simulink model "PMSM"  (R2020a)
settings: Solver=ode45  StartTime=0.0  StopTime=10.0  RelTol=1e-6  AbsTol=1e-8
values from neighbouring files (symbols this model uses):
  B = 0.08    [Mainprog.m]
  Ba = alphas * Jhat - Bhat    (= 0.17)    [Mainprog.m]
  J = 0.05*0.25    (= 0.0125)    [Mainprog.m]
  kis = alphas * (Bhat + Ba)    (= 5)    [Mainprog.m]
  kps = alphas * Jhat    (= 0.25)    [Mainprog.m]
  np = 2    [Mainprog.m]
  Rs = 1.33    [Mainprog.m]
undefined symbols (not defined in the file or in its folder): Beta_initial, Beta_timeup, fluxm, fluxm_hat, i, I_rated, isd0, isq0, j, kicd, kicq, kpcd, kpcq, Lsd, Lsd_hat, Lsq, Lsq_hat, Rad, Raq, Speed_initial, Speed_timeup, Speed_valueup, T_extra_timeup, T_extra_valup, T_ref1_timeup, T_ref1_valup, T_ref2_timeup, T_ref2_valup, thetar0, usd0, usq0, VconvLim, wr0, ws
settings Model: ExtModeTrigMode=oneshot  ExtModeArmWhenConnect=off  ExtModeAutoUpdateStatusClock=off  Creator=e6zebra  LastModifiedBy=miche
settings SolverCC: AutoScaleAbsTol=off
settings DataIOCC: SaveFormat=Array  SignalLoggingSaveFormat=ModelDataLogs  ReturnWorkspaceOutputs=off
settings OptimizationCC: BlockReduction=off  BooleanDataType=off  ExpressionDepthLimit=2147483647  InitFltsAndDblsToZero=on  LifeSpan=inf
settings DebuggingCC: SaveWithParameterizedLinksMsg=none  UnderspecifiedInitializationDetection=Classic  MergeDetectMultiDrivingBlocksExec=none  SignalResolutionControl=TryResolveAllWithWarning  MultiTaskDSMMsg=warning  MultiTaskCondExecSysMsg=none  FcnCallInpInsideContextMsg=warning  StateNameClashWarn=warning  SFUnexpectedBacktrackingDiag=warning  SFNoUnconditionalDefaultTransitionDiag=warning  SFExecutionAtInitializationDiag=none  ArithmeticOperatorsInVariantConditions=warning
settings HardwareCC: ProdBitPerPointer=32  ProdBitPerSizeT=32  ProdBitPerPtrDiffT=32  ProdLargestAtomicFloat=None  ProdIntDivRoundTo=Undefined  ProdEndianess=Unspecified  ProdWordSize=32  ProdHWDeviceType=32-bit Generic  TargetUnknown=on
settings ModelReferenceCC: PropagateSignalLabelsOutOfModel=off
settings SFSimCC: SimUseLocalCustomCode=off  CustomCodeUndefinedFunction=UseInterfaceOnly
settings RTWCC: TemplateMakefile=grt.tmf  RTWUseLocalCustomCode=off
settings CodeAppCC: StateflowObjectComments=on
settings GRTTargetCC: TargetFcnLib=ansi_tfl_tmw.mat  TargetLangStandard=C89/C90 (ANSI)  CombineOutputUpdateFcns=off  GRTInterface=on
settings ConfigComp: CovMetricSettings=dw  CovHtmlReporting=on  CovSaveCumulativeToWorkspaceVar=on  CovSaveSingleToWorkspaceVar=on  CovExternalEMLEnable=off  CovSFcnEnable=off

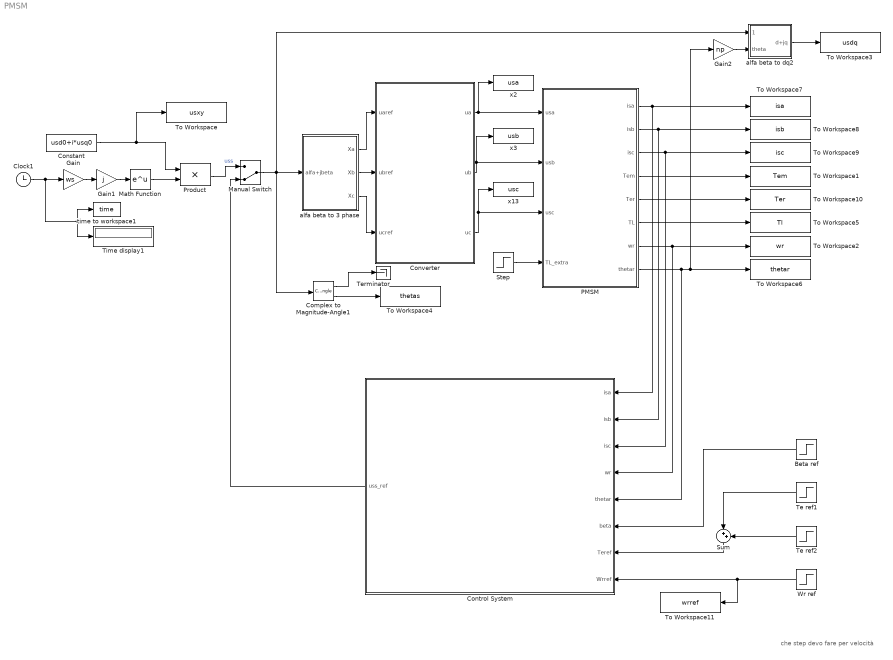
== system PMSM ==
  note: che step devo fare per velocità
  Beta ref : Step  Time=Beta_timeup  Before=Beta_initial  After=Beta_initial  SampleTime=0
  Clock1 : Clock
  Complex to Magnitude-Angle1 : ComplexToMagnitudeAngle
  Constant : Constant  Value=usd0+i*usq0
  Control System : Subsystem
  Converter : Subsystem
  Gain : Gain  Gain=ws
  Gain1 : Gain  Gain=j  SaturateOnIntegerOverflow=on  OutDataTypeStr=Inherit: Same as input  ParamDataTypeStr=Inherit: Same as input
  Gain2 : Gain  Gain=np
  Manual Switch : ManualSwitch  CurrentSetting=0
  Math Function : Math  SignedPower=on  SaturateOnIntegerOverflow=on
  PMSM : Subsystem
  Product : Product  SaturateOnIntegerOverflow=on  OutDataTypeStr=Inherit: Same as first input
  Step : Step  Time=T_extra_timeup  After=T_extra_valup  SampleTime=0
  Sum : Sum  Inputs=|++
  Te ref1 : Step  Time=T_ref1_timeup  After=T_ref1_valup  SampleTime=0
  Te ref2 : Step  Time=T_ref2_timeup  After=T_ref2_valup  SampleTime=0
  Terminator : Terminator
  Time display1 : Display
  To Workspace : ToWorkspace  VariableName=usxy  SampleTime=-1
  To Workspace1 : ToWorkspace  VariableName=Tem  SampleTime=-1
  To Workspace10 : ToWorkspace  VariableName=Ter  SampleTime=-1
  To Workspace11 : ToWorkspace  VariableName=wrref  SampleTime=-1
  To Workspace2 : ToWorkspace  VariableName=wr  SampleTime=-1
  To Workspace3 : ToWorkspace  VariableName=usdq  SampleTime=-1
  To Workspace4 : ToWorkspace  VariableName=thetas  SampleTime=-1
  To Workspace5 : ToWorkspace  VariableName=Tl  SampleTime=-1
  To Workspace6 : ToWorkspace  VariableName=thetar  SampleTime=-1
  To Workspace7 : ToWorkspace  VariableName=isa  SampleTime=-1
  To Workspace8 : ToWorkspace  VariableName=isb  SampleTime=-1
  To Workspace9 : ToWorkspace  VariableName=isc  SampleTime=-1
  Wr ref : Step  Time=Speed_timeup  Before=Speed_initial  After=Speed_valueup  SampleTime=0
  alfa beta to 3 phase : Subsystem
  alfa beta to dq2 : Subsystem
  time to workspace1 : ToWorkspace  VariableName=time  SampleTime=-1
  x13 : ToWorkspace  VariableName=usc  SampleTime=-1
  x2 : ToWorkspace  VariableName=usa  SampleTime=-1
  x3 : ToWorkspace  VariableName=usb  SampleTime=-1
  wires:
  Converter/1(ua) -> x2/1, PMSM/1(usa)
  alfa beta to 3 phase/3(Xc) -> Converter/3(ucref)
  Complex to Magnitude-Angle1/2 -> To Workspace4/1
  alfa beta to 3 phase/1(Xa) -> Converter/1(uaref)
  Gain1/1 -> Math Function/1
  Clock1/1 -> Time display1/1, time to workspace1/1, Gain/1
  alfa beta to 3 phase/2(Xb) -> Converter/2(ubref)
  Gain/1 -> Gain1/1
  Math Function/1 -> Product/2
  Complex to Magnitude-Angle1/1 -> Terminator/1
  Step/1 -> PMSM/4(TL_extra)
  Constant/1 -> To Workspace/1, Product/1
  alfa beta to dq2/1(d+jq) -> To Workspace3/1
  PMSM/8(thetar) -> Control System/5(thetar), To Workspace6/1, Gain2/1
  Gain2/1 -> alfa beta to dq2/2(theta)
  PMSM/7(wr) -> To Workspace2/1, Control System/4(wr)
  PMSM/6(TL) -> To Workspace5/1
  Converter/2(ub) -> x3/1, PMSM/2(usb)
  Converter/3(uc) -> PMSM/3(usc), x13/1
  PMSM/1(isa) -> To Workspace7/1, Control System/1(isa)
  PMSM/2(isb) -> To Workspace8/1, Control System/2(isb)
  PMSM/3(isc) -> To Workspace9/1, Control System/3(isc)
  PMSM/4(Tem) -> To Workspace1/1
  PMSM/5(Ter) -> To Workspace10/1
  Manual Switch/1 -> Complex to Magnitude-Angle1/1, alfa beta to dq2/1(alfa+jbeta), alfa beta to 3 phase/1(alfa+jbeta)
  Product/1 -> Manual Switch/1  "uss"
  Control System/1(uss_ref) -> Manual Switch/2
  Te ref1/1 -> Sum/1
  Te ref2/1 -> Sum/2
  Sum/1 -> Control System/7(Teref)
  Wr ref/1 -> To Workspace11/1, Control System/8(Wrref)
  Beta ref/1 -> Control System/6(beta)

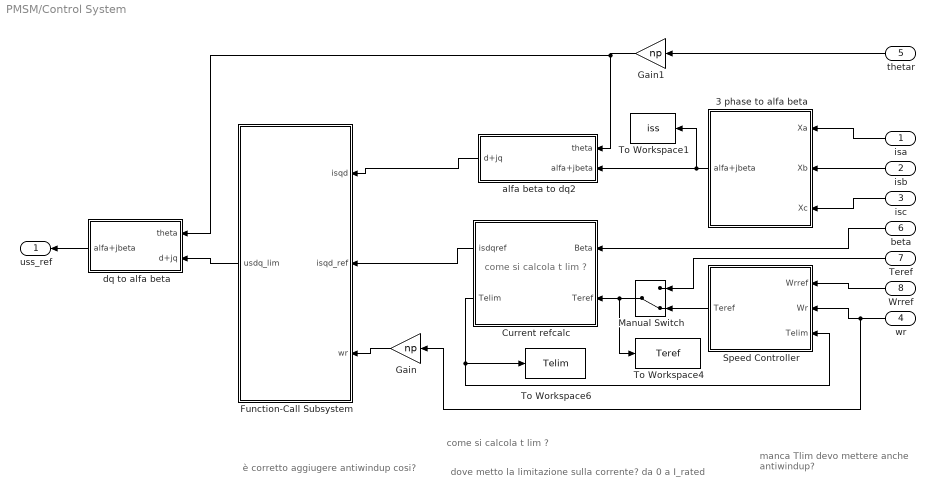
== system PMSM/Control System ==
  note: come si calcola t lim ?
  note: dove metto la limitazione sulla corrente? da 0 a I_rated
  note: è corretto aggiugere antiwindup cosi?
  note: manca Tlim
      |
      | devo mettere anche antiwindup?
  note: come si calcola t lim ?
  isa : Inport
  isb : Inport  Port=2
  isc : Inport  Port=3
  wr : Inport  Port=4
  thetar : Inport  Port=5
  beta : Inport  Port=6
  Teref : Inport  Port=7
  Wrref : Inport  Port=8
  3 phase to alfa beta : Subsystem
  Current refcalc : Subsystem
  Function-Call Subsystem : Subsystem  TreatAsAtomicUnit=on
  Gain : Gain  Gain=np
  Gain1 : Gain  Gain=np
  Manual Switch : ManualSwitch  CurrentSetting=0
  Speed Controller : Subsystem
  To Workspace1 : ToWorkspace  VariableName=iss  SampleTime=-1
  To Workspace4 : ToWorkspace  VariableName=Teref  SampleTime=-1
  To Workspace6 : ToWorkspace  VariableName=Telim  SampleTime=-1
  alfa beta to dq2 : Subsystem
  dq to alfa beta : Subsystem
  uss_ref : Outport
  wires:
  dq to alfa beta/1(alfa+jbeta) -> uss_ref/1
  alfa beta to dq2/1(d+jq) -> Function-Call Subsystem/1(isqd)
  3 phase to alfa beta/1(alfa+jbeta) -> To Workspace1/1, alfa beta to dq2/2(alfa+jbeta)
  Speed Controller/1(Teref) -> Manual Switch/2
  Manual Switch/1 -> To Workspace4/1, Current refcalc/2(Teref)
  Wrref/1 -> Speed Controller/1(Wrref)
  Teref/1 -> Manual Switch/1
  beta/1 -> Current refcalc/1(Beta)
  isc/1 -> 3 phase to alfa beta/3(Xc)
  isb/1 -> 3 phase to alfa beta/2(Xb)
  isa/1 -> 3 phase to alfa beta/1(Xa)
  Current refcalc/1(isdqref) -> Function-Call Subsystem/2(isqd_ref)
  thetar/1 -> Gain1/1
  wr/1 -> Gain/1, Speed Controller/2(Wr)
  Current refcalc/2(Telim) -> To Workspace6/1, Speed Controller/3(Telim)
  Gain1/1 -> alfa beta to dq2/1(theta), dq to alfa beta/1(theta)
  Gain/1 -> Function-Call Subsystem/3(wr)
  Function-Call Subsystem/1(usdq_lim) -> dq to alfa beta/2(d+jq)

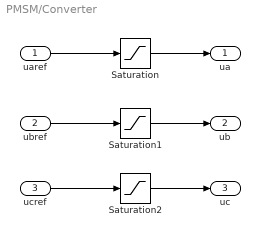
== system PMSM/Converter ==
  uaref : Inport
  ubref : Inport  Port=2
  ucref : Inport  Port=3
  Saturation : Saturate  UpperLimit=VconvLim  LowerLimit=-VconvLim
  Saturation1 : Saturate  UpperLimit=VconvLim  LowerLimit=-VconvLim
  Saturation2 : Saturate  UpperLimit=VconvLim  LowerLimit=-VconvLim
  ua : Outport  VectorParamsAs1DForOutWhenUnconnected=off
  ub : Outport  Port=2  VectorParamsAs1DForOutWhenUnconnected=off
  uc : Outport  Port=3  VectorParamsAs1DForOutWhenUnconnected=off
  wires:
  Saturation2/1 -> uc/1
  Saturation1/1 -> ub/1
  Saturation/1 -> ua/1
  uaref/1 -> Saturation/1
  ubref/1 -> Saturation1/1
  ucref/1 -> Saturation2/1

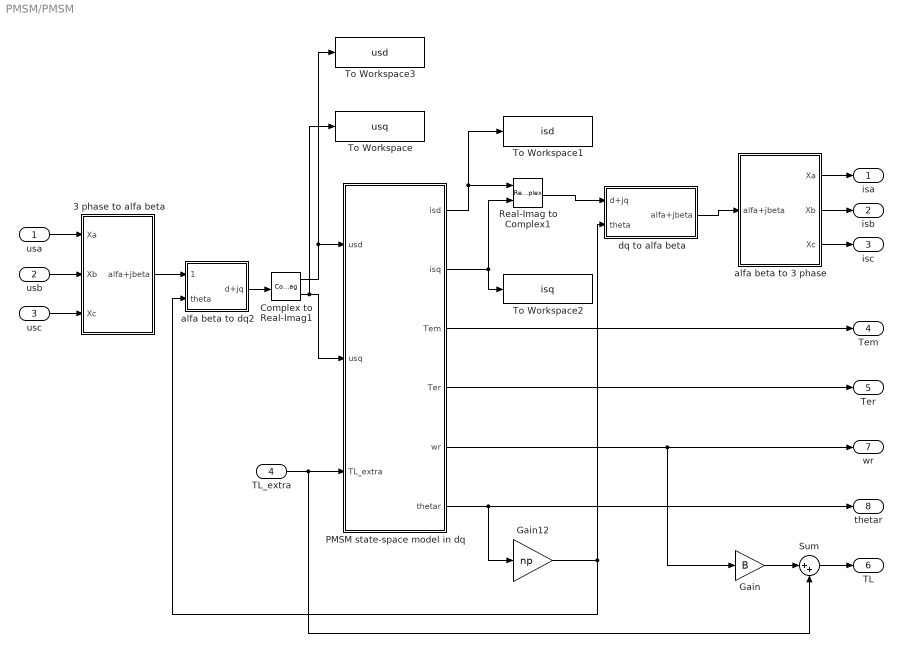
== system PMSM/PMSM ==
  usa : Inport
  usb : Inport  Port=2
  usc : Inport  Port=3
  TL_extra : Inport  Port=4
  3 phase to alfa beta : Subsystem
  Complex to Real-Imag1 : ComplexToRealImag
  Gain : Gain  Gain=B
  Gain12 : Gain  Gain=np
  PMSM state-space model in dq : Subsystem
  Real-Imag to Complex1 : RealImagToComplex
  Sum : Sum  Inputs=|++
  To Workspace : ToWorkspace  VariableName=usq  SampleTime=-1
  To Workspace1 : ToWorkspace  VariableName=isd  SampleTime=-1
  To Workspace2 : ToWorkspace  VariableName=isq  SampleTime=-1
  To Workspace3 : ToWorkspace  VariableName=usd  SampleTime=-1
  alfa beta to 3 phase : Subsystem
  alfa beta to dq2 : Subsystem
  dq to alfa beta : Subsystem
  isa : Outport
  isb : Outport  Port=2
  isc : Outport  Port=3
  Tem : Outport  Port=4
  Ter : Outport  Port=5
  TL : Outport  Port=6
  wr : Outport  Port=7
  thetar : Outport  Port=8
  wires:
  usb/1 -> 3 phase to alfa beta/2(Xb)
  usa/1 -> 3 phase to alfa beta/1(Xa)
  usc/1 -> 3 phase to alfa beta/3(Xc)
  3 phase to alfa beta/1(alfa+jbeta) -> alfa beta to dq2/1(alfa+jbeta)
  alfa beta to dq2/1(d+jq) -> Complex to Real-Imag1/1
  Complex to Real-Imag1/1 -> To Workspace3/1, PMSM state-space model in dq/1(usd)
  Complex to Real-Imag1/2 -> PMSM state-space model in dq/2(usq), To Workspace/1
  TL_extra/1 -> PMSM state-space model in dq/3(TL_extra), Sum/2
  PMSM state-space model in dq/1(isd) -> To Workspace1/1, Real-Imag to Complex1/1
  PMSM state-space model in dq/2(isq) -> To Workspace2/1, Real-Imag to Complex1/2
  alfa beta to 3 phase/1(Xa) -> isa/1
  alfa beta to 3 phase/2(Xb) -> isb/1
  alfa beta to 3 phase/3(Xc) -> isc/1
  PMSM state-space model in dq/5(wr) -> wr/1, Gain/1
  dq to alfa beta/1(alfa+jbeta) -> alfa beta to 3 phase/1(alfa+jbeta)
  Real-Imag to Complex1/1 -> dq to alfa beta/1(d+jq)
  PMSM state-space model in dq/6(thetar) -> thetar/1, Gain12/1
  Gain/1 -> Sum/1
  Sum/1 -> TL/1
  PMSM state-space model in dq/4(Ter) -> Ter/1
  PMSM state-space model in dq/3(Tem) -> Tem/1
  Gain12/1 -> dq to alfa beta/2(theta), alfa beta to dq2/2(theta)

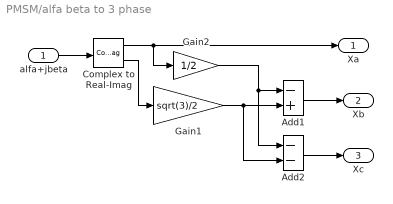
== system PMSM/alfa beta to 3 phase ==
  alfa+jbeta : Inport
  Add1 : Sum  Inputs=-+
  Add2 : Sum  Inputs=--
  Complex to Real-Imag : ComplexToRealImag
  Gain1 : Gain  Gain=sqrt(3)/2
  Gain2 : Gain  Gain=1/2
  Xa : Outport  VectorParamsAs1DForOutWhenUnconnected=off
  Xb : Outport  Port=2  VectorParamsAs1DForOutWhenUnconnected=off
  Xc : Outport  Port=3  VectorParamsAs1DForOutWhenUnconnected=off
  wires:
  alfa+jbeta/1 -> Complex to Real-Imag/1
  Complex to Real-Imag/1 -> Xa/1, Gain2/1
  Add2/1 -> Xc/1
  Add1/1 -> Xb/1
  Complex to Real-Imag/2 -> Gain1/1
  Gain1/1 -> Add1/2, Add2/2
  Gain2/1 -> Add1/1, Add2/1

== system PMSM/alfa beta to dq2 ==
  alfa+jbeta : Inport
  theta : Inport  Port=2
  Gain : Gain  Gain=-j  SaturateOnIntegerOverflow=on  OutDataTypeStr=Inherit: Same as input  ParamDataTypeStr=Inherit: Same as input
  Math Function : Math  SignedPower=on  SaturateOnIntegerOverflow=on
  Product : Product  SaturateOnIntegerOverflow=on  OutDataTypeStr=Inherit: Same as first input
  d+jq : Outport  VectorParamsAs1DForOutWhenUnconnected=off
  wires:
  theta/1 -> Gain/1
  Gain/1 -> Math Function/1
  Math Function/1 -> Product/2
  alfa+jbeta/1 -> Product/1
  Product/1 -> d+jq/1

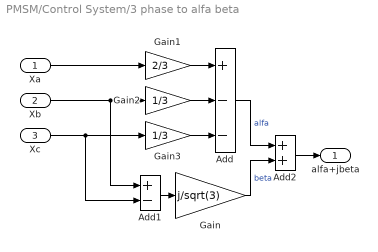
== system PMSM/Control System/3 phase to alfa beta ==
  Xa : Inport
  Xb : Inport  Port=2
  Xc : Inport  Port=3
  Add : Sum  Inputs=+--
  Add1 : Sum  Inputs=+-
  Add2 : Sum
  Gain : Gain  Gain=j/sqrt(3)
  Gain1 : Gain  Gain=2/3
  Gain2 : Gain  Gain=1/3
  Gain3 : Gain  Gain=1/3
  alfa+jbeta : Outport  VectorParamsAs1DForOutWhenUnconnected=off
  wires:
  Add1/1 -> Gain/1
  Add2/1 -> alfa+jbeta/1
  Gain/1 -> Add2/2  "beta"
  Add/1 -> Add2/1  "alfa"
  Gain3/1 -> Add/3
  Gain2/1 -> Add/2
  Gain1/1 -> Add/1
  Xa/1 -> Gain1/1
  Xb/1 -> Gain2/1, Add1/1
  Xc/1 -> Gain3/1, Add1/2

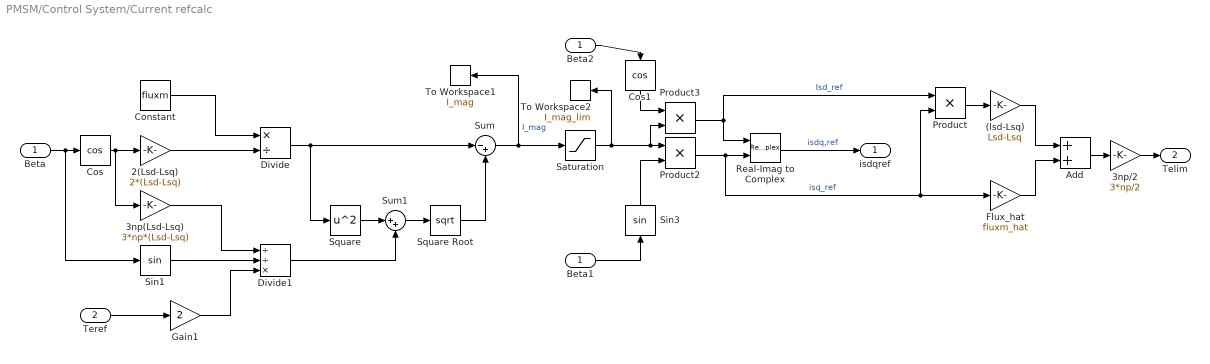
== system PMSM/Control System/Current refcalc ==
  Beta : Inport
  Teref : Inport  Port=2
  (lsd-Lsq) : Gain  Gain=Lsd-Lsq
  2(Lsd-Lsq) : Gain  Gain=2*(Lsd-Lsq)
  3np(Lsd-Lsq) : Gain  Gain=3*np*(Lsd-Lsq)
  3np/2 : Gain  Gain=3*np/2
  Add : Sum
  Beta1 : InportShadow
  Beta2 : InportShadow
  Constant : Constant  Value=fluxm
  Cos : Trigonometry  Operator=cos
  Cos1 : Trigonometry  Operator=cos
  Divide : Product  Inputs=*/
  Divide1 : Product  Inputs=//*
  Flux_hat : Gain  Gain=fluxm_hat
  Gain1 : Gain  Gain=2
  Product : Product
  Product2 : Product
  Product3 : Product
  Real-Imag to Complex : RealImagToComplex
  Saturation : Saturate  UpperLimit=I_rated*sqrt(2)  LowerLimit=0
  Sin1 : Trigonometry
  Sin3 : Trigonometry
  Square : Math  Operator=square  SaturateOnIntegerOverflow=on
  Square Root : Sqrt  SaturateOnIntegerOverflow=on
  Sum : Sum  Inputs=|-+
  Sum1 : Sum  Inputs=|++
  To Workspace1 : ToWorkspace  VariableName=I_mag  SampleTime=-1
  To Workspace2 : ToWorkspace  VariableName=I_mag_lim  SampleTime=-1
  isdqref : Outport
  Telim : Outport  Port=2
  wires:
  Cos/1 -> 3np(Lsd-Lsq)/1, 2(Lsd-Lsq)/1
  2(Lsd-Lsq)/1 -> Divide/2
  Constant/1 -> Divide/1
  Divide/1 -> Sum/1, Square/1
  Square/1 -> Sum1/1
  Divide1/1 -> Sum1/2
  Sum1/1 -> Square Root/1
  Square Root/1 -> Sum/2
  Beta/1 -> Sin1/1, Cos/1
  3np(Lsd-Lsq)/1 -> Divide1/1
  Sin1/1 -> Divide1/2
  Gain1/1 -> Divide1/3
  Teref/1 -> Gain1/1
  Sum/1 -> To Workspace1/1, Saturation/1  "I_mag"
  Saturation/1 -> To Workspace2/1, Product3/2, Product2/1
  Real-Imag to Complex/1 -> isdqref/1  "isdq,ref"
  Product2/1 -> Product/2, Flux_hat/1, Real-Imag to Complex/2  "isq_ref"
  Product3/1 -> Product/1, Real-Imag to Complex/1  "Isd_ref"
  Cos1/1 -> Product3/1
  Sin3/1 -> Product2/2
  3np/2/1 -> Telim/1
  Add/1 -> 3np/2/1
  Product/1 -> (lsd-Lsq)/1
  Flux_hat/1 -> Add/2
  (lsd-Lsq)/1 -> Add/1
  Beta1/1 -> Sin3/1
  Beta2/1 -> Cos1/1

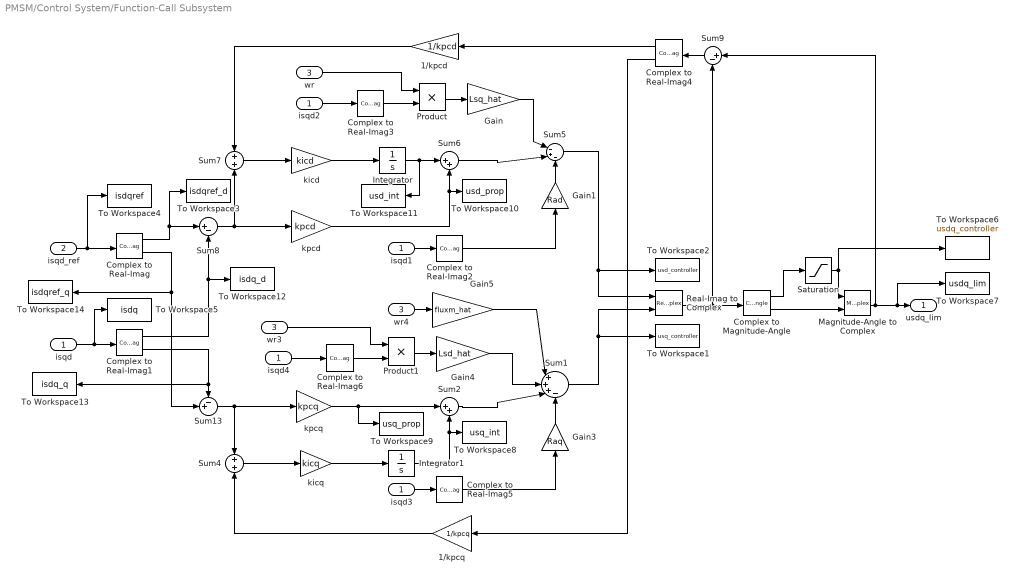
== system PMSM/Control System/Function-Call Subsystem ==
  isqd : Inport
  isqd_ref : Inport  Port=2
  wr : Inport  Port=3
  1/kpcd : Gain  Gain=1/kpcd
  1/kpcq : Gain  Gain=1/kpcq
  Complex to Magnitude-Angle : ComplexToMagnitudeAngle
  Complex to Real-Imag : ComplexToRealImag
  Complex to Real-Imag1 : ComplexToRealImag
  Complex to Real-Imag2 : ComplexToRealImag  Output=Real
  Complex to Real-Imag3 : ComplexToRealImag  Output=Imag
  Complex to Real-Imag4 : ComplexToRealImag
  Complex to Real-Imag5 : ComplexToRealImag  Output=Imag
  Complex to Real-Imag6 : ComplexToRealImag  Output=Real
  Gain : Gain  Gain=Lsq_hat
  Gain1 : Gain  Gain=Rad
  Gain3 : Gain  Gain=Raq
  Gain4 : Gain  Gain=Lsd_hat
  Gain5 : Gain  Gain=fluxm_hat
  Integrator : Integrator
  Integrator1 : Integrator
  Magnitude-Angle to Complex : MagnitudeAngleToComplex
  Product : Product
  Product1 : Product
  Real-Imag to Complex : RealImagToComplex
  Saturation : Saturate  UpperLimit=VconvLim  LowerLimit=-VconvLim
  Sum1 : Sum  Inputs=|+++-
  Sum13 : Sum  Inputs=-+|
  Sum2 : Sum  Inputs=|++
  Sum4 : Sum
  Sum5 : Sum  Inputs=|-+-
  Sum6 : Sum  Inputs=|++
  Sum7 : Sum
  Sum8 : Sum  Inputs=|+-
  Sum9 : Sum  Inputs=|+-
  To Workspace1 : ToWorkspace  VariableName=usq_controller  SampleTime=-1
  To Workspace10 : ToWorkspace  VariableName=usd_prop  SampleTime=-1
  To Workspace11 : ToWorkspace  VariableName=usd_int  SampleTime=-1
  To Workspace12 : ToWorkspace  VariableName=isdq_d  SampleTime=-1
  To Workspace13 : ToWorkspace  VariableName=isdq_q  SampleTime=-1
  To Workspace14 : ToWorkspace  VariableName=isdqref_q  SampleTime=-1
  To Workspace2 : ToWorkspace  VariableName=usd_controller  SampleTime=-1
  To Workspace3 : ToWorkspace  VariableName=isdqref_d  SampleTime=-1
  To Workspace4 : ToWorkspace  VariableName=isdqref  SampleTime=-1
  To Workspace5 : ToWorkspace  VariableName=isdq  SampleTime=-1
  To Workspace6 : ToWorkspace  VariableName=usdq_controller  SampleTime=-1
  To Workspace7 : ToWorkspace  VariableName=usdq_lim  SampleTime=-1
  To Workspace8 : ToWorkspace  VariableName=usq_int  SampleTime=-1
  To Workspace9 : ToWorkspace  VariableName=usq_prop  SampleTime=-1
  isqd{1..4} (4 alike) : InportShadow
  kicd : Gain  Gain=kicd
  kicq : Gain  Gain=kicq
  kpcd : Gain  Gain=kpcd
  kpcq : Gain  Gain=kpcq
  wr3 : InportShadow  Port=3
  wr4 : InportShadow  Port=3
  usdq_lim : Outport
  wires:
  Complex to Real-Imag4/2 -> 1/kpcq/1
  wr4/1 -> Gain5/1
  Integrator1/1 -> Sum2/2, To Workspace8/1
  kicd/1 -> Integrator/1
  Integrator/1 -> To Workspace11/1, Sum6/1
  Complex to Magnitude-Angle/2 -> Magnitude-Angle to Complex/2
  Complex to Real-Imag/2 -> To Workspace14/1, Sum13/2
  Saturation/1 -> To Workspace6/1, Magnitude-Angle to Complex/1
  isqd3/1 -> Complex to Real-Imag5/1
  Complex to Real-Imag3/1 -> Product/2
  Sum4/1 -> kicq/1
  Gain/1 -> Sum5/1
  isqd_ref/1 -> To Workspace4/1, Complex to Real-Imag/1
  Complex to Real-Imag1/1 -> Sum8/2, To Workspace12/1
  isqd4/1 -> Complex to Real-Imag6/1
  Gain5/1 -> Sum1/1
  Complex to Real-Imag2/1 -> Gain1/1
  wr/1 -> Product/1
  Product/1 -> Gain/1
  isqd1/1 -> Complex to Real-Imag2/1
  Gain3/1 -> Sum1/4
  Sum5/1 -> Real-Imag to Complex/1, To Workspace2/1
  Sum8/1 -> kpcd/1, Sum7/2
  Sum9/1 -> Complex to Real-Imag4/1
  Complex to Real-Imag4/1 -> 1/kpcd/1
  Gain1/1 -> Sum5/3
  Sum1/1 -> Real-Imag to Complex/2, To Workspace1/1
  Sum13/1 -> Sum4/1, kpcq/1
  Complex to Real-Imag6/1 -> Product1/2
  wr3/1 -> Product1/1
  Complex to Real-Imag1/2 -> To Workspace13/1, Sum13/1
  Product1/1 -> Gain4/1
  isqd2/1 -> Complex to Real-Imag3/1
  Complex to Real-Imag/1 -> To Workspace3/1, Sum8/1
  kpcd/1 -> To Workspace10/1, Sum6/2
  1/kpcq/1 -> Sum4/2
  Sum7/1 -> kicd/1
  1/kpcd/1 -> Sum7/1
  Complex to Real-Imag5/1 -> Gain3/1
  kpcq/1 -> Sum2/1, To Workspace9/1
  Real-Imag to Complex/1 -> Complex to Magnitude-Angle/1, Sum9/2
  kicq/1 -> Integrator1/1
  Magnitude-Angle to Complex/1 -> Sum9/1, To Workspace7/1, usdq_lim/1
  Gain4/1 -> Sum1/2
  Sum2/1 -> Sum1/3
  isqd/1 -> To Workspace5/1, Complex to Real-Imag1/1
  Complex to Magnitude-Angle/1 -> Saturation/1
  Sum6/1 -> Sum5/2

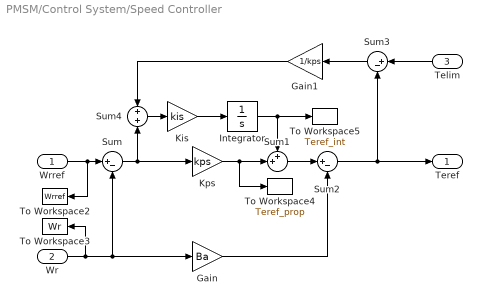
== system PMSM/Control System/Speed Controller ==
  Wrref : Inport
  Wr : Inport  Port=2
  Telim : Inport  Port=3
  Gain : Gain  Gain=Ba
  Gain1 : Gain  Gain=1/kps
  Integrator : Integrator
  Kis : Gain  Gain=kis
  Kps : Gain  Gain=kps
  Sum : Sum  Inputs=|+-
  Sum1 : Sum  Inputs=++|
  Sum2 : Sum  Inputs=|+-
  Sum3 : Sum  Inputs=|+-
  Sum4 : Sum
  To Workspace2 : ToWorkspace  VariableName=Wrref  SampleTime=-1
  To Workspace3 : ToWorkspace  VariableName=Wr  SampleTime=-1
  To Workspace4 : ToWorkspace  VariableName=Teref_prop  SampleTime=-1
  To Workspace5 : ToWorkspace  VariableName=Teref_int  SampleTime=-1
  Teref : Outport
  wires:
  Kps/1 -> To Workspace4/1, Sum1/2
  Wrref/1 -> To Workspace2/1, Sum/1
  Sum/1 -> Sum4/2, Kps/1
  Wr/1 -> To Workspace3/1, Gain/1, Sum/2
  Sum1/1 -> Sum2/1
  Gain/1 -> Sum2/2
  Sum2/1 -> Sum3/2, Teref/1
  Telim/1 -> Sum3/1
  Sum3/1 -> Gain1/1
  Sum4/1 -> Kis/1
  Gain1/1 -> Sum4/1
  Kis/1 -> Integrator/1
  Integrator/1 -> To Workspace5/1, Sum1/1

== system PMSM/Control System/alfa beta to dq2 ==
  theta : Inport
  alfa+jbeta : Inport  Port=2
  Gain : Gain  Gain=-j  SaturateOnIntegerOverflow=on  OutDataTypeStr=Inherit: Same as input  ParamDataTypeStr=Inherit: Same as input
  Math Function : Math  SignedPower=on  SaturateOnIntegerOverflow=on
  Product : Product  SaturateOnIntegerOverflow=on  OutDataTypeStr=Inherit: Same as first input
  d+jq : Outport  VectorParamsAs1DForOutWhenUnconnected=off
  wires:
  theta/1 -> Gain/1
  Gain/1 -> Math Function/1
  Math Function/1 -> Product/2
  alfa+jbeta/1 -> Product/1
  Product/1 -> d+jq/1

== system PMSM/Control System/dq to alfa beta ==
  theta : Inport
  d+jq : Inport  Port=2
  Gain : Gain  Gain=j  SaturateOnIntegerOverflow=on  OutDataTypeStr=Inherit: Same as input  ParamDataTypeStr=Inherit: Same as input
  Math Function : Math  SignedPower=on  SaturateOnIntegerOverflow=on
  Product : Product  SaturateOnIntegerOverflow=on  OutDataTypeStr=Inherit: Same as first input
  alfa+jbeta : Outport
  wires:
  theta/1 -> Gain/1
  Gain/1 -> Math Function/1
  Math Function/1 -> Product/2
  d+jq/1 -> Product/1
  Product/1 -> alfa+jbeta/1

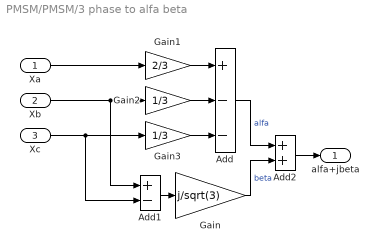
== system PMSM/PMSM/3 phase to alfa beta ==
  Xa : Inport
  Xb : Inport  Port=2
  Xc : Inport  Port=3
  Add : Sum  Inputs=+--
  Add1 : Sum  Inputs=+-
  Add2 : Sum
  Gain : Gain  Gain=j/sqrt(3)
  Gain1 : Gain  Gain=2/3
  Gain2 : Gain  Gain=1/3
  Gain3 : Gain  Gain=1/3
  alfa+jbeta : Outport  VectorParamsAs1DForOutWhenUnconnected=off
  wires:
  Add1/1 -> Gain/1
  Add2/1 -> alfa+jbeta/1
  Gain/1 -> Add2/2  "beta"
  Add/1 -> Add2/1  "alfa"
  Gain3/1 -> Add/3
  Gain2/1 -> Add/2
  Gain1/1 -> Add/1
  Xa/1 -> Gain1/1
  Xb/1 -> Gain2/1, Add1/1
  Xc/1 -> Gain3/1, Add1/2

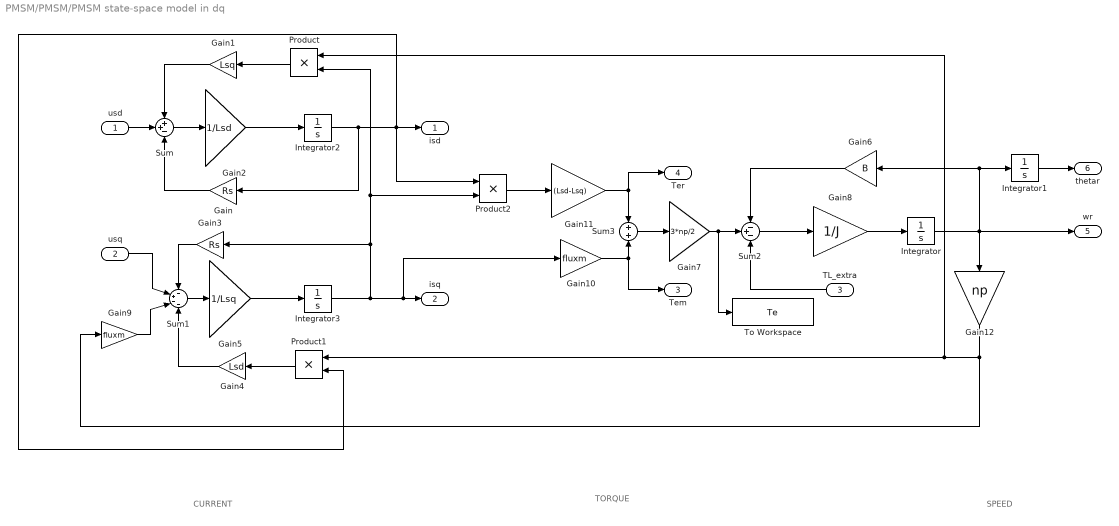
== system PMSM/PMSM/PMSM state-space model in dq ==
  note: SPEED
  note: TORQUE
  note: CURRENT
  usd : Inport
  usq : Inport  Port=2
  TL_extra : Inport  Port=3
  Gain : Gain  Gain=Rs
  Gain1 : Gain  Gain=Lsq
  Gain10 : Gain  Gain=fluxm
  Gain11 : Gain  Gain=(Lsd-Lsq)
  Gain12 : Gain  Gain=np
  Gain2 : Gain  Gain=1/Lsd
  Gain3 : Gain  Gain=Rs
  Gain4 : Gain  Gain=Lsd
  Gain5 : Gain  Gain=1/Lsq
  Gain6 : Gain  Gain=B
  Gain7 : Gain  Gain=3*np/2
  Gain8 : Gain  Gain=1/J
  Gain9 : Gain  Gain=fluxm
  Integrator : Integrator  InitialCondition=wr0
  Integrator1 : Integrator  InitialCondition=thetar0
  Integrator2 : Integrator  InitialCondition=isd0
  Integrator3 : Integrator  InitialCondition=isq0
  Product : Product
  Product1 : Product
  Product2 : Product
  Sum : Sum  Inputs=++-
  Sum1 : Sum  Inputs=-+--
  Sum2 : Sum  Inputs=-+-
  Sum3 : Sum
  To Workspace : ToWorkspace  VariableName=Te  SampleTime=-1
  isd : Outport
  isq : Outport  Port=2
  Tem : Outport  Port=3
  Ter : Outport  Port=4
  wr : Outport  Port=5
  thetar : Outport  Port=6
  wires:
  usd/1 -> Sum/2
  Product/1 -> Gain1/1
  Sum/1 -> Gain2/1
  Gain2/1 -> Integrator2/1
  Product1/1 -> Gain4/1
  Integrator3/1 -> Gain10/1, isq/1, Product2/2, Product/2, Gain3/1
  usq/1 -> Sum1/2
  Sum1/1 -> Gain5/1
  Gain5/1 -> Integrator3/1
  TL_extra/1 -> Sum2/3
  Gain6/1 -> Sum2/1
  Gain8/1 -> Integrator/1
  Sum2/1 -> Gain8/1
  Gain9/1 -> Sum1/3
  Integrator1/1 -> thetar/1
  Sum3/1 -> Gain7/1
  Gain7/1 -> To Workspace/1, Sum2/2
  Gain10/1 -> Tem/1, Sum3/2
  Product2/1 -> Gain11/1
  Gain11/1 -> Ter/1, Sum3/1
  Gain3/1 -> Sum1/1
  Gain4/1 -> Sum1/4
  Integrator2/1 -> isd/1, Product2/1, Product1/2, Gain/1
  Integrator/1 -> Gain12/1, wr/1, Integrator1/1, Gain6/1
  Gain/1 -> Sum/3
  Gain1/1 -> Sum/1
  Gain12/1 -> Gain9/1, Product/1, Product1/1

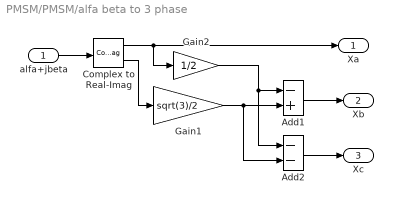
== system PMSM/PMSM/alfa beta to 3 phase ==
  alfa+jbeta : Inport
  Add1 : Sum  Inputs=-+
  Add2 : Sum  Inputs=--
  Complex to Real-Imag : ComplexToRealImag
  Gain1 : Gain  Gain=sqrt(3)/2
  Gain2 : Gain  Gain=1/2
  Xa : Outport  VectorParamsAs1DForOutWhenUnconnected=off
  Xb : Outport  Port=2  VectorParamsAs1DForOutWhenUnconnected=off
  Xc : Outport  Port=3  VectorParamsAs1DForOutWhenUnconnected=off
  wires:
  alfa+jbeta/1 -> Complex to Real-Imag/1
  Complex to Real-Imag/1 -> Xa/1, Gain2/1
  Add2/1 -> Xc/1
  Add1/1 -> Xb/1
  Complex to Real-Imag/2 -> Gain1/1
  Gain1/1 -> Add1/2, Add2/2
  Gain2/1 -> Add1/1, Add2/1

== system PMSM/PMSM/alfa beta to dq2 ==
  alfa+jbeta : Inport
  theta : Inport  Port=2
  Gain : Gain  Gain=-j  SaturateOnIntegerOverflow=on  OutDataTypeStr=Inherit: Same as input  ParamDataTypeStr=Inherit: Same as input
  Math Function : Math  SignedPower=on  SaturateOnIntegerOverflow=on
  Product : Product  SaturateOnIntegerOverflow=on  OutDataTypeStr=Inherit: Same as first input
  d+jq : Outport  VectorParamsAs1DForOutWhenUnconnected=off
  wires:
  theta/1 -> Gain/1
  Gain/1 -> Math Function/1
  Math Function/1 -> Product/2
  alfa+jbeta/1 -> Product/1
  Product/1 -> d+jq/1

== system PMSM/PMSM/dq to alfa beta ==
  d+jq : Inport
  theta : Inport  Port=2
  Gain : Gain  Gain=j  SaturateOnIntegerOverflow=on  OutDataTypeStr=Inherit: Same as input  ParamDataTypeStr=Inherit: Same as input
  Math Function : Math  SignedPower=on  SaturateOnIntegerOverflow=on
  Product : Product  SaturateOnIntegerOverflow=on  OutDataTypeStr=Inherit: Same as first input
  alfa+jbeta : Outport
  wires:
  theta/1 -> Gain/1
  Gain/1 -> Math Function/1
  Math Function/1 -> Product/2
  d+jq/1 -> Product/1
  Product/1 -> alfa+jbeta/1
